simulink model "simulink_proyecto"  (R2025a)
settings: Solver=VariableStepAuto  StartTime=0.0  StopTime=30  RelTol=1e-3
libraries: cstblocks x8
settings Model: Creator=danielsaenzobando  LastModifiedBy=danielsaenzobando

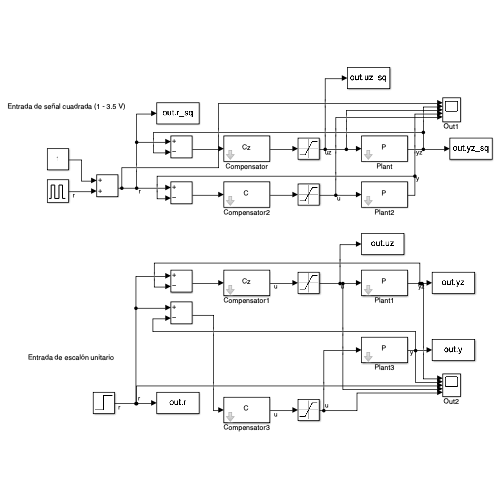
[thumbnail: Simulink's stored preview of the top-level diagram]
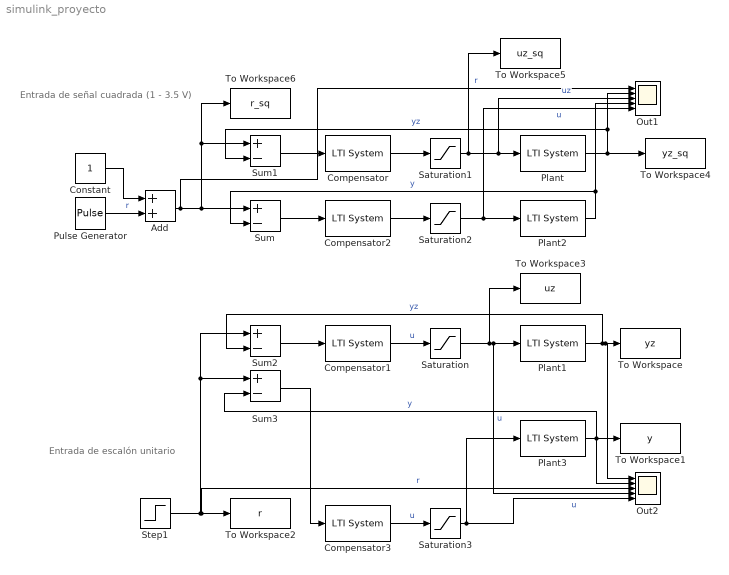
== system simulink_proyecto ==
  note: Entrada de señal cuadrada (1 - 3.5 V)
  note: Entrada de escalón unitario
  Add : Sum
  Compensator : cstblocks/LTI System  sys=Cz  IC=[]  PadeOrder=0
  Compensator1 : cstblocks/LTI System  sys=Cz  IC=[]  PadeOrder=0
  Compensator2 : cstblocks/LTI System  sys=C  IC=[]  PadeOrder=0
  Compensator3 : cstblocks/LTI System  sys=C  IC=[]  PadeOrder=0
  Constant : Constant
  Out1 : Scope  NumInputPorts=5
      settings: ActiveDisplayYMinimum=-2.37366085485109  ActiveDisplayYMaximum=6.81326009594375
  Out2 : Scope  NumInputPorts=5
      settings: ActiveDisplayYMinimum=-0.21170464018731866  ActiveDisplayYMaximum=1.9053417616858686
  Plant{,1..3} (4 alike) : cstblocks/LTI System  sys=P  IC=[]  PadeOrder=0
  Pulse Generator : DiscretePulseGenerator  PulseType=Time based  Amplitude=2.5  Period=12  PulseWidth=50  PhaseDelay=6
  Saturation{,1..3} (4 alike) : Saturate  UpperLimit=5  LowerLimit=0
  Step1 : Step  Time=0  SampleTime=0
  Sum{,1..3} (4 alike) : Sum  Inputs=+-
  To Workspace : ToWorkspace  VariableName=yz  SaveFormat=Timeseries  SampleTime=-1
  To Workspace1 : ToWorkspace  VariableName=y  SaveFormat=Timeseries  SampleTime=-1
  To Workspace2 : ToWorkspace  VariableName=r  SaveFormat=Timeseries  SampleTime=-1
  To Workspace3 : ToWorkspace  VariableName=uz  SaveFormat=Timeseries  SampleTime=-1
  To Workspace4 : ToWorkspace  VariableName=yz_sq  SaveFormat=Timeseries  SampleTime=-1
  To Workspace5 : ToWorkspace  VariableName=uz_sq  SaveFormat=Timeseries  SampleTime=-1
  To Workspace6 : ToWorkspace  VariableName=r_sq  SaveFormat=Timeseries  SampleTime=-1
  wires:
  Plant3/1 -> Out2/2, Sum3/2, To Workspace1/1  "y"
  Plant/1 -> Out1/2, Sum1/2, To Workspace4/1  "yz"
  Saturation/1 -> Plant1/1, Out2/4, To Workspace3/1  "u"
  Saturation2/1 -> Plant2/1, Out1/5  "u"
  Saturation3/1 -> Plant3/1, Out2/5  "u"
  Saturation1/1 -> Plant/1, Out1/3, To Workspace5/1  "uz"
  Compensator1/1 -> Saturation/1  "u"
  Compensator2/1 -> Saturation2/1
  Compensator/1 -> Saturation1/1
  Sum3/1 -> Compensator3/1
  Sum/1 -> Compensator2/1
  Step1/1 -> Out2/3, To Workspace2/1, Sum2/1, Sum3/1  "r"
  Add/1 -> Sum/1, To Workspace6/1, Sum1/1, Out1/1  "r"
  Plant2/1 -> Out1/4, Sum/2  "y"
  Sum2/1 -> Compensator1/1
  Compensator3/1 -> Saturation3/1  "u"
  Pulse Generator/1 -> Add/2  "r"
  Sum1/1 -> Compensator/1
  Plant1/1 -> Out2/1, To Workspace/1, Sum2/2  "yz"
  Constant/1 -> Add/1
